simulink model "GFLIB_Limit_BAM_F32"  (Simulink 8.3)
settings: Solver=ode45  StartTime=0.0  StopTime=10.0  RelTol=1e-3
undefined symbols (not defined in the file): f32LowerLim, f32UpperLimit
settings Model: Creator=B17364  LastModifiedBy=B17364
settings OptimizationCC: ExpressionDepthLimit=2147483647
settings DebuggingCC: FcnCallInpInsideContextMsg=UseLocalSettings  StrictBusMsg=Warning

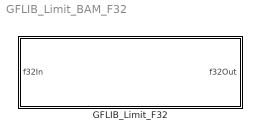
== system GFLIB_Limit_BAM_F32 ==
  GFLIB_Limit_F32 : Subsystem  mask(GFLIB_Limit){f32UpperLimit=f32UpperLimit, f32LowerLim=f32LowerLim}
      mask help: Bit accurate model of the GFLIB_Limit function.
      mask init:
      | pos = get_param(gcb, 'Position');width = pos(3) - pos(1); height = pos(4) - pos(2);tX=width/2;tY=height*0.9;
      mask Display: color('black');port_label('input',1,'f32In');port_label('output',1,'f32Out');color('black');disp('GFLIB_Limit_F32');color('blue');text(tX,tY, 'BAM', 'horizontalAlignment', 'center');

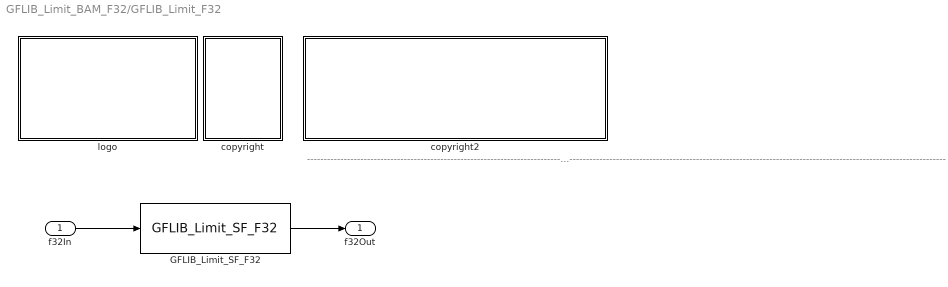
== system GFLIB_Limit_BAM_F32/GFLIB_Limit_F32 ==
  note: ---------------------------------------------------------------------------------------------------------------------------------------------------------------------------------------------------
  f32In : Inport
  GFLIB_Limit_SF_F32 : S-Function  FunctionName=GFLIB_Limit_SF_F32  Parameters=f32UpperLimit,f32LowerLim  EnableBusSupport=off
  copyright : Subsystem
      mask Display:
      | text(10,90,'FILE:');text(10,75,'DESRIPTION:')
      | text(10,60,'COPYRIGHT:')
      | text(10,45,'VERSION:')
      | text(10,30,'DATE:')
      | text(10,15,'AUTHOR:')
  copyright2 : Subsystem
      mask Display:
      | text(10,90,'GFLIB_Limit_BAM_F32.mdl');text(10,75,'Limit function');text(10,60,'Freescale')
      | text(10,45,'0.1');text(10,30,'03-Jul-2011');text(10,15,'');
  logo : Subsystem
      mask Display: image(imread('logo.jpg'))
  f32Out : Outport
  wires:
  f32In/1 -> GFLIB_Limit_SF_F32/1
  GFLIB_Limit_SF_F32/1 -> f32Out/1

== system GFLIB_Limit_BAM_F32/GFLIB_Limit_F32/copyright ==

== system GFLIB_Limit_BAM_F32/GFLIB_Limit_F32/copyright2 ==

== system GFLIB_Limit_BAM_F32/GFLIB_Limit_F32/logo ==
